simulink model "wheel_vel_model"  (R2015a)
settings: Solver=ode3  StartTime=0  StopTime=5  RelTol=1e-3
settings Model: Creator=BML  LastModifiedBy=BML
settings SolverCC: AutoInsertRateTranBlk=on

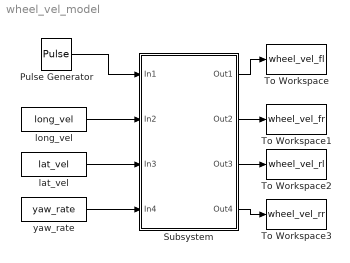
== system wheel_vel_model ==
  Pulse Generator : DiscretePulseGenerator  PulseType=Time based  Amplitude=0  Period=8  PulseWidth=5  PhaseDelay=3
  Subsystem : Subsystem
  To Workspace : ToWorkspace  VariableName=wheel_vel_fl  SaveFormat=Timeseries
  To Workspace1 : ToWorkspace  VariableName=wheel_vel_fr  SaveFormat=Timeseries
  To Workspace2 : ToWorkspace  VariableName=wheel_vel_rl  SaveFormat=Timeseries
  To Workspace3 : ToWorkspace  VariableName=wheel_vel_rr  SaveFormat=Timeseries
  lat_vel : FromWorkspace  VariableName=lat_vel  SampleTime=0
  long_vel : FromWorkspace  VariableName=long_vel  SampleTime=0
  yaw_rate : FromWorkspace  VariableName=yaw_rate  SampleTime=0
  wires:
  Pulse Generator/1 -> Subsystem/1(In1)
  long_vel/1 -> Subsystem/2(In2)
  lat_vel/1 -> Subsystem/3(In3)
  yaw_rate/1 -> Subsystem/4(In4)
  Subsystem/1(Out1) -> To Workspace/1
  Subsystem/2(Out2) -> To Workspace1/1
  Subsystem/3(Out3) -> To Workspace2/1
  Subsystem/4(Out4) -> To Workspace3/1

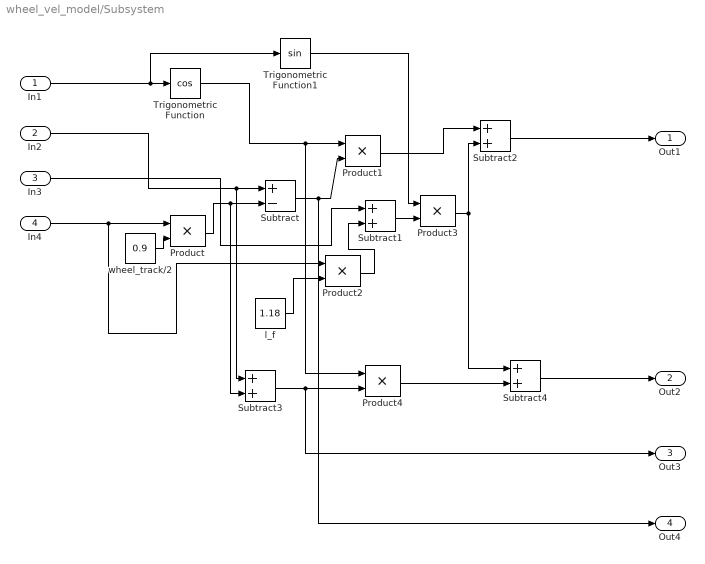
== system wheel_vel_model/Subsystem ==
  In1 : Inport
  In2 : Inport  Port=2
  In3 : Inport  Port=3
  In4 : Inport  Port=4
  Product{,1..4} (5 alike) : Product
  Subtract : Sum  Inputs=+-
  Subtract{1..4} (4 alike) : Sum
  Trigonometric Function : Trigonometry  Operator=cos
  Trigonometric Function1 : Trigonometry
  l_f : Constant  Value=1.18
  wheel_track/2 : Constant  Value=0.9
  Out1 : Outport
  Out2 : Outport  Port=2
  Out3 : Outport  Port=3
  Out4 : Outport  Port=4
  wires:
  In2/1 -> Subtract3/1, Subtract/1
  l_f/1 -> Product2/2
  Subtract3/1 -> Out3/1, Product4/2
  Trigonometric Function/1 -> Product4/1, Product1/1
  Subtract1/1 -> Product3/2
  Subtract/1 -> Out4/1, Product1/2
  Product4/1 -> Subtract4/2
  Subtract4/1 -> Out2/1
  In3/1 -> Subtract1/1
  Product/1 -> Subtract3/2, Subtract/2
  Product2/1 -> Subtract1/2
  Product1/1 -> Subtract2/1
  In4/1 -> Product/1, Product2/1
  wheel_track/2/1 -> Product/2
  Trigonometric Function1/1 -> Product3/1
  Subtract2/1 -> Out1/1
  In1/1 -> Trigonometric Function1/1, Trigonometric Function/1
  Product3/1 -> Subtract2/2, Subtract4/1
